simulink model "ex4"  (R2020a)
settings: Solver=VariableStepAuto  StartTime=0.0  StopTime=10.0  RelTol=1e-3
values from neighbouring files (symbols this model uses):
  C = [0 1/(L*C)]    [Rezolvare.m]
  L = 100    [Rezolvare.m]
  R = 1000    [Rezolvare.m]

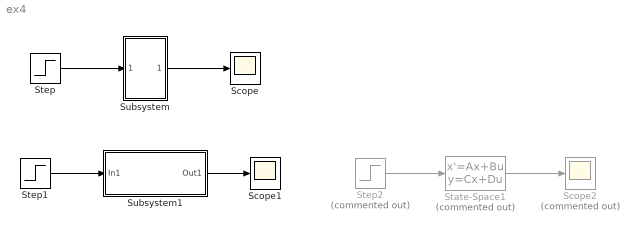
== system ex4 ==
  Scope : Scope
  Scope1 : Scope
  Scope2 : Scope  Commented=on
  State-Space1 : StateSpace  Commented=on  A=[R/L 1/(L*C); 1 0]  B=[1;0]  C=[0 1/(L*C)]  D=[0 0; 0 0]  InitialCondition=0
  Step : Step  SampleTime=0
  Step1 : Step  SampleTime=0
  Step2 : Step  Commented=on  SampleTime=0
  Subsystem : Subsystem  mask{R=10000, C=0.0001}
      mask prompts: R "R="; C "C="
  Subsystem1 : Subsystem  mask{R=10000, L=100, C=0.0001}
      mask prompts: R "R="; L "L="; C "C="
  wires:
  Step/1 -> Subsystem/1(In1)
  Subsystem/1(Out1) -> Scope/1
  State-Space1/1 -> Scope2/1
  Step2/1 -> State-Space1/1
  Step1/1 -> Subsystem1/1(In1)
  Subsystem1/1(Out1) -> Scope1/1

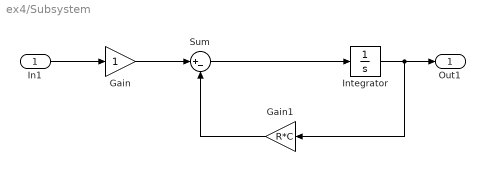
== system ex4/Subsystem ==
  In1 : Inport
  Gain : Gain
  Gain1 : Gain  Gain=R*C
  Integrator : Integrator
  Sum : Sum  Inputs=|+-
  Out1 : Outport
  wires:
  Gain/1 -> Sum/1
  Integrator/1 -> Out1/1, Gain1/1
  Gain1/1 -> Sum/2
  Sum/1 -> Integrator/1
  In1/1 -> Gain/1

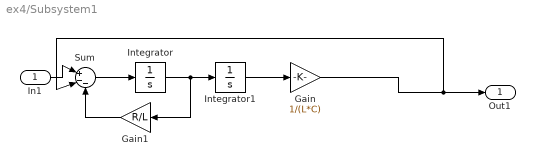
== system ex4/Subsystem1 ==
  In1 : Inport
  Gain : Gain  Gain=1/(L*C)
  Gain1 : Gain  Gain=R/L
  Integrator : Integrator
  Integrator1 : Integrator
  Sum : Sum  Inputs=|+--
  Out1 : Outport
  wires:
  In1/1 -> Sum/1
  Sum/1 -> Integrator/1
  Integrator/1 -> Gain1/1, Integrator1/1
  Integrator1/1 -> Gain/1
  Gain/1 -> Sum/2, Out1/1
  Gain1/1 -> Sum/3
